simulink model "Double_mass_damper_system"  (R2023b)
settings: Solver=ode4  StartTime=0.0  StopTime=10.0  FixedStep=0.01  RelTol=1e-3
settings Model: Creator=Santhosh  LastModifiedBy=Santhosh

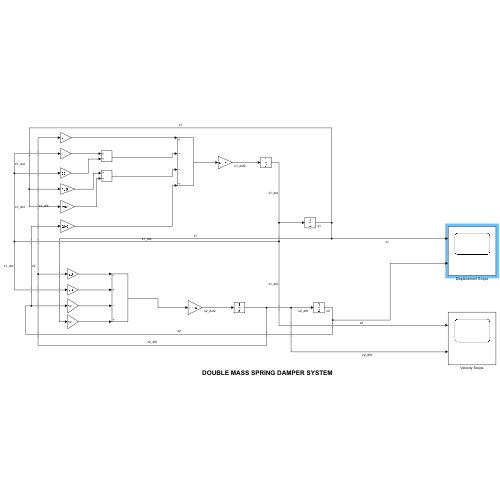
[thumbnail: Simulink's stored preview of the top-level diagram]
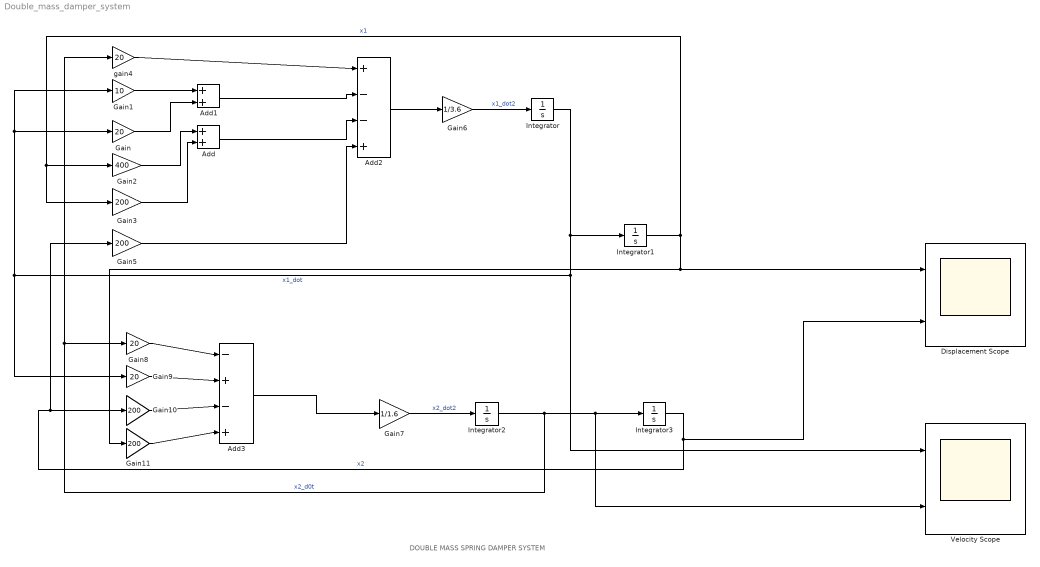
== system Double_mass_damper_system ==
  note: DOUBLE MASS SPRING DAMPER SYSTEM
  Add : Sum
  Add1 : Sum
  Add2 : Sum  Inputs=+||-||-||+
  Add3 : Sum  Inputs=-||+||-||+
  Displacement Scope : Scope  NumInputPorts=2
  Gain : Gain  Gain=20
  Gain1 : Gain  Gain=10
  Gain{3,5,10..11} (4 alike) : Gain  Gain=200
  Gain2 : Gain  Gain=400
  Gain6 : Gain  Gain=1/3.6
  Gain7 : Gain  Gain=1/1.6
  Gain8 : Gain  Gain=20
  Gain9 : Gain  Gain=20
  Integrator : Integrator
  Integrator1 : Integrator  InitialCondition=0.05
  Integrator2 : Integrator
  Integrator3 : Integrator  InitialCondition=0.05
  Velocity Scope : Scope  NumInputPorts=2
  gain4 : Gain  Gain=20
  wires:
  Integrator/1 -> Velocity Scope/1, Gain9/1, Gain/1, Gain1/1, Integrator1/1  "x1_dot"
  Gain1/1 -> Add1/1
  Gain/1 -> Add1/2
  Gain2/1 -> Add/1
  Gain3/1 -> Add/2
  Integrator2/1 -> Velocity Scope/2, Integrator3/1, Gain8/1, gain4/1  "x2_d0t"
  Gain5/1 -> Add2/4
  Integrator1/1 -> Gain11/1, Displacement Scope/1, Gain3/1, Gain2/1  "x1"
  Add/1 -> Add2/3
  gain4/1 -> Add2/1
  Add1/1 -> Add2/2
  Add2/1 -> Gain6/1
  Gain6/1 -> Integrator/1  "x1_dot2"
  Gain7/1 -> Integrator2/1  "x2_dot2"
  Gain11/1 -> Add3/4
  Gain10/1 -> Add3/3
  Gain9/1 -> Add3/2
  Gain8/1 -> Add3/1
  Integrator3/1 -> Displacement Scope/2, Gain5/1, Gain10/1  "x2"
  Add3/1 -> Gain7/1
